simulink model "I_P_control_model_right"  (R2015b)
settings: Solver=VariableStepAuto  StartTime=0.0  StopTime=203  RelTol=1e-3
values from neighbouring files (symbols this model uses):
  a0 = 0.0424941737179    [I_P_control_right.mat]
  a1 = 0.246207630573    [I_P_control_right.mat]
  b0 = 0.047154360386    [I_P_control_right.mat]
  ki = 0.038    [I_P_control_right.mat]
  kp = 0.1775    [I_P_control_right.mat]
  r = 1    [I_P_control_right.mat]
  sample_time = 1    [I_P_control_right.mat]
settings Model: Creator=ryodo  LastModifiedBy=ryodo

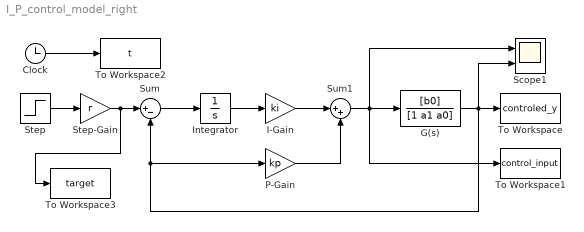
== system I_P_control_model_right ==
  Clock : Clock
  G(s) : TransferFcn  Numerator=[b0]  Denominator=[1 a1 a0]
  I-Gain : Gain  Gain=ki
  Integrator : Integrator
  P-Gain : Gain  Gain=kp
  Scope1 : Scope  NumInputPorts=2
  Step : Step  Time=0  SampleTime=sample_time
  Step-Gain : Gain  Gain=r
  Sum : Sum  Inputs=|+-
  Sum1 : Sum  Inputs=|++
  To Workspace : ToWorkspace  VariableName=controled_y  SampleTime=sample_time
  To Workspace1 : ToWorkspace  VariableName=control_input  SampleTime=sample_time
  To Workspace2 : ToWorkspace  VariableName=t  SampleTime=sample_time
  To Workspace3 : ToWorkspace  VariableName=target  SampleTime=-1
  wires:
  G(s)/1 -> Scope1/2, To Workspace/1, Sum/2, P-Gain/1
  Sum1/1 -> Scope1/1, To Workspace1/1, G(s)/1
  I-Gain/1 -> Sum1/1
  Integrator/1 -> I-Gain/1
  Sum/1 -> Integrator/1
  P-Gain/1 -> Sum1/2
  Step/1 -> Step-Gain/1
  Step-Gain/1 -> To Workspace3/1, Sum/1
  Clock/1 -> To Workspace2/1
